simulink model "modelo_completo"  (R2020a)
settings: Solver=FixedStepAuto  StartTime=0.0  StopTime=1000.0  FixedStep=sampleTime  RelTol=1e-3
values from neighbouring files (symbols this model uses):
  FIR = [0 ... (first row only)    [Lab_3.m]
  G = 0    [Lab_3.m]
  mu = 0.03    [Lab_3.m]
  sampleTime = 0.03    [Lab_3.m]
undefined symbols (not defined in the file or in its folder): magnitude
settings Model: Creator=Gaming  LastModifiedBy=Duarte
settings SFSimCC: CustomCodeUndefinedFunction=UseInterfaceOnly

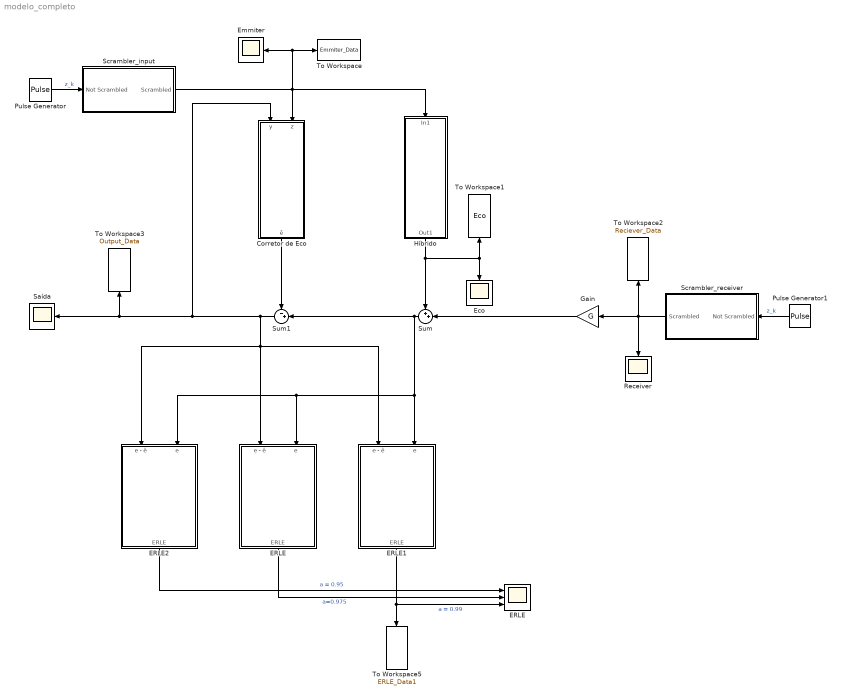
== system modelo_completo ==
  Corretor de Eco : Subsystem
  ERLE : Subsystem
  "ERLE " : Scope  NumInputPorts=3
  ERLE1 : Subsystem
  ERLE2 : Subsystem
  Eco : Scope
  Emmiter : Scope
  Gain : Gain  Gain=G
  Híbrido : Subsystem
  Pulse Generator : DiscretePulseGenerator  SampleTime=sampleTime
  Pulse Generator1 : DiscretePulseGenerator  SampleTime=sampleTime
  Receiver : Scope
  Saída : Scope
  Scrambler_input : Subsystem
  Scrambler_receiver : Subsystem
  Sum : Sum  Inputs=++|
  Sum1 : Sum  Inputs=-+|
  To Workspace : ToWorkspace  VariableName=Emmiter_Data  SaveFormat=Structure With Time  SampleTime=-1
  To Workspace1 : ToWorkspace  VariableName=Eco  SaveFormat=Structure With Time  SampleTime=-1
  To Workspace2 : ToWorkspace  VariableName=Reciever_Data  SaveFormat=Structure With Time  SampleTime=-1
  To Workspace3 : ToWorkspace  VariableName=Output_Data  SaveFormat=Structure With Time  SampleTime=-1
  To Workspace5 : ToWorkspace  VariableName=ERLE_Data1  SaveFormat=Structure With Time  SampleTime=-1
  wires:
  Pulse Generator1/1 -> Scrambler_receiver/1(Not Scrambled)  "z_k"
  Scrambler_receiver/1(Scrambled) -> Receiver/1, To Workspace2/1, Gain/1
  Gain/1 -> Sum/2
  Pulse Generator/1 -> Scrambler_input/1(Not Scrambled)  "z_k"
  Scrambler_input/1(Scrambled) -> To Workspace/1, Emmiter/1, Híbrido/1(In1), Corretor de Eco/2(z)
  Corretor de Eco/1(ê) -> Sum1/1
  Sum1/1 -> Saída/1, To Workspace3/1, Corretor de Eco/1(y), ERLE2/1(e - ê), ERLE/1(e - ê), ERLE1/1(e - ê)
  ERLE/1(ERLE) -> "ERLE "/2  "a=0.975"
  Híbrido/1(Out1) -> To Workspace1/1, Eco/1, Sum/1
  ERLE1/1(ERLE) -> "ERLE "/3, To Workspace5/1  "a = 0.99"
  ERLE2/1(ERLE) -> "ERLE "/1  "a = 0.95"
  Sum/1 -> Sum1/2, ERLE2/2(e), ERLE/2(e), ERLE1/2(e)

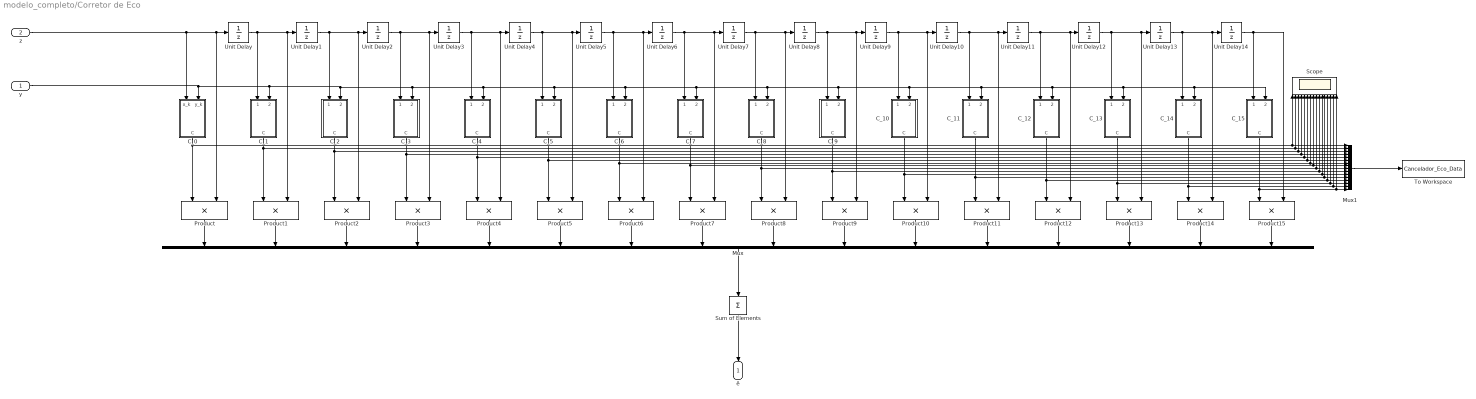
== system modelo_completo/Corretor de Eco ==
  y : Inport
  z : Inport  Port=2
  C_0 : Subsystem
  C_1 : Subsystem
  C_10 : Subsystem
  C_11 : Subsystem
  C_12 : Subsystem
  C_13 : Subsystem
  C_14 : Subsystem
  C_15 : Subsystem
  C_2 : Subsystem
  C_3 : Subsystem
  C_4 : Subsystem
  C_5 : Subsystem
  C_6 : Subsystem
  C_7 : Subsystem
  C_8 : Subsystem
  C_9 : Subsystem
  Mux : Mux  Inputs=16
  Mux1 : Mux  Inputs=16
  Product{,1..15} (16 alike) : Product
  Scope : Scope  NumInputPorts=16
  Sum of Elements : Sum  Inputs=+
  To Workspace : ToWorkspace  VariableName=Cancelador_Eco_Data  SaveFormat=Structure With Time  SampleTime=-1
  Unit Delay{,1..14} (15 alike) : UnitDelay  SampleTime=-1  HasFrameUpgradeWarning=on
  ê : Outport  VectorParamsAs1DForOutWhenUnconnected=off
  wires:
  Unit Delay9/1 -> C_10/1(x_k+1), Unit Delay10/1, Product10/2
  Unit Delay6/1 -> C_7/1(x_k+1), Unit Delay7/1, Product7/2
  C_14/1(C) -> Mux1/15, Scope/15, Product14/1
  Unit Delay8/1 -> C_9/1(x_k+1), Unit Delay9/1, Product9/2
  Product1/1 -> Mux/2
  C_13/1(C) -> Mux1/14, Scope/14, Product13/1
  Unit Delay3/1 -> C_4/1(x_k+1), Unit Delay4/1, Product4/2
  Unit Delay/1 -> Unit Delay1/1, Product1/2, C_1/1(x_k+1)
  Product13/1 -> Mux/14
  C_10/1(C) -> Mux1/11, Scope/11, Product10/1
  Unit Delay1/1 -> C_2/1(x_k+1), Unit Delay2/1, Product2/2
  Unit Delay7/1 -> C_8/1(x_k+1), Unit Delay8/1, Product8/2
  Unit Delay4/1 -> C_5/1(x_k+1), Unit Delay5/1, Product5/2
  C_9/1(C) -> Mux1/10, Scope/10, Product9/1
  Unit Delay13/1 -> C_14/1(x_k+1), Unit Delay14/1, Product14/2
  Unit Delay12/1 -> C_13/1(x_k+1), Unit Delay13/1, Product13/2
  C_11/1(C) -> Mux1/12, Scope/12, Product11/1
  Product6/1 -> Mux/7
  Unit Delay10/1 -> C_11/1(x_k+1), Unit Delay11/1, Product11/2
  C_0/1(C) -> Product/1, Mux1/1, Scope/1
  z/1 -> Unit Delay/1, Product/2, C_0/1(x_k)
  C_6/1(C) -> Mux1/7, Scope/7, Product6/1
  Unit Delay11/1 -> C_12/1(x_k+1), Unit Delay12/1, Product12/2
  C_3/1(C) -> Product3/1, Mux1/4, Scope/4
  Product15/1 -> Mux/16
  C_2/1(C) -> Product2/1, Mux1/3, Scope/3
  C_4/1(C) -> Mux1/5, Scope/5, Product4/1
  Unit Delay2/1 -> C_3/1(x_k+1), Unit Delay3/1, Product3/2
  Product4/1 -> Mux/5
  Mux/1 -> Sum of Elements/1
  Product3/1 -> Mux/4
  C_7/1(C) -> Product7/1, Mux1/8, Scope/8
  Product14/1 -> Mux/15
  Product5/1 -> Mux/6
  Product9/1 -> Mux/10
  C_1/1(C) -> Mux1/2, Scope/2, Product1/1
  Unit Delay5/1 -> C_6/1(x_k+1), Unit Delay6/1, Product6/2
  Product7/1 -> Mux/8
  Product12/1 -> Mux/13
  Product8/1 -> Mux/9
  C_8/1(C) -> Mux1/9, Scope/9, Product8/1
  Product11/1 -> Mux/12
  Product10/1 -> Mux/11
  C_15/1(C) -> Mux1/16, Scope/16, Product15/1
  Unit Delay14/1 -> C_15/1(x_k+1), Product15/2
  C_12/1(C) -> Product12/1, Mux1/13, Scope/13
  Sum of Elements/1 -> ê/1
  Product/1 -> Mux/1
  Product2/1 -> Mux/3
  Mux1/1 -> To Workspace/1
  y/1 -> C_0/2(y_k), C_7/2(y_k+1), C_11/2(y_k+1), C_14/2(y_k+1), C_15/2(y_k+1), C_13/2(y_k+1), C_12/2(y_k+1), C_10/2(y_k+1), C_9/2(y_k+1), C_8/2(y_k+1), C_6/2(y_k+1), C_5/2(y_k+1), C_4/2(y_k+1), C_3/2(y_k+1), C_2/2(y_k+1), C_1/2(y_k+1)
  C_5/1(C) -> Product5/1, Mux1/6, Scope/6

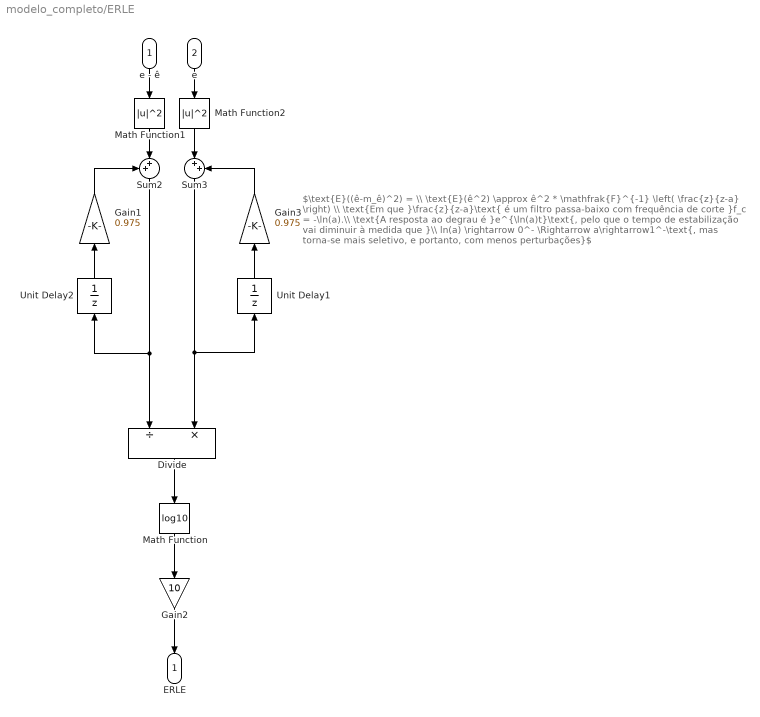
== system modelo_completo/ERLE ==
  note: $\text{E}((ê-m_ê)^2) = \\ \text{E}(ê^2) \approx ê^2 * \mathfrak{F}^{-1} \left( \frac{z}{z-a} \right) \\ \text{Em que }\frac{z}{z-a}\text{ é um filtro passa-baixo com frequência de corte }f_c = -\ln(a).\\ \text{A resposta ao degrau é }e^{\ln(a)t}\text{, pelo que o tempo de estabilização vai diminuir à medida que }\\ ln(a) \rightarrow 0^- \Rightarrow a\rightarrow1^-\text{, mas torna-se mais seletivo, e portanto, com menos perturbações}$
  e - ê : Inport
  e : Inport  Port=2
  Divide : Product  Inputs=/*
  Gain1 : Gain  Gain=0.975
  Gain2 : Gain  Gain=10
  Gain3 : Gain  Gain=0.975
  Math Function : Math  Operator=log10  SignedPower=on  SaturateOnIntegerOverflow=on
  Math Function1 : Math  Operator=magnitude^2  SignedPower=on  SaturateOnIntegerOverflow=on
  Math Function2 : Math  Operator=magnitude^2  SignedPower=on  SaturateOnIntegerOverflow=on
  Sum2 : Sum  Inputs=++|
  Sum3 : Sum  Inputs=|++
  Unit Delay1 : UnitDelay  SampleTime=-1  HasFrameUpgradeWarning=on
  Unit Delay2 : UnitDelay  SampleTime=-1  HasFrameUpgradeWarning=on
  ERLE : Outport  VectorParamsAs1DForOutWhenUnconnected=off
  wires:
  Math Function2/1 -> Sum3/1
  Math Function/1 -> Gain2/1
  Divide/1 -> Math Function/1
  Unit Delay2/1 -> Gain1/1
  Unit Delay1/1 -> Gain3/1
  e - ê/1 -> Math Function1/1
  Sum3/1 -> Divide/2, Unit Delay1/1
  Gain3/1 -> Sum3/2
  Math Function1/1 -> Sum2/2
  Sum2/1 -> Unit Delay2/1, Divide/1
  Gain1/1 -> Sum2/1
  e/1 -> Math Function2/1
  Gain2/1 -> ERLE/1

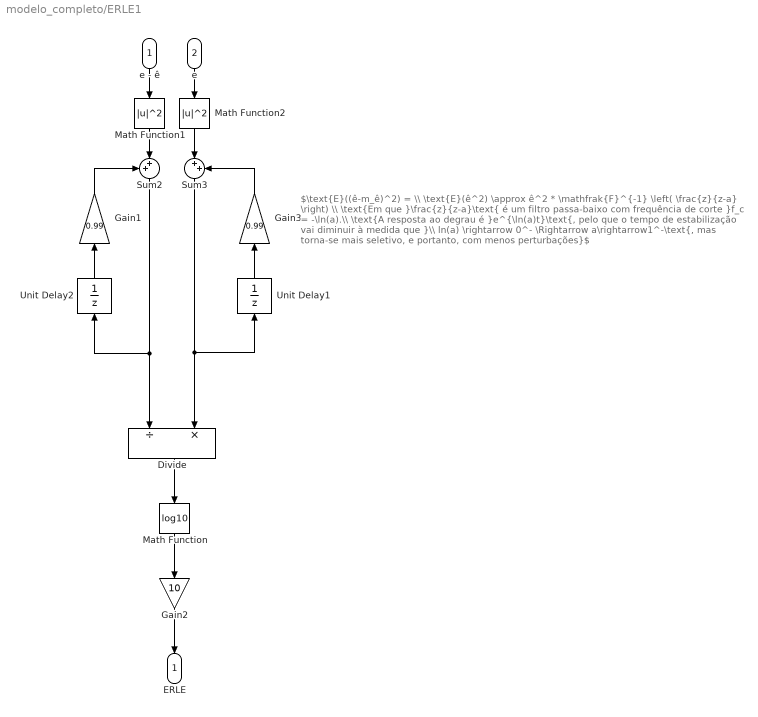
== system modelo_completo/ERLE1 ==
  note: $\text{E}((ê-m_ê)^2) = \\ \text{E}(ê^2) \approx ê^2 * \mathfrak{F}^{-1} \left( \frac{z}{z-a} \right) \\ \text{Em que }\frac{z}{z-a}\text{ é um filtro passa-baixo com frequência de corte }f_c = -\ln(a).\\ \text{A resposta ao degrau é }e^{\ln(a)t}\text{, pelo que o tempo de estabilização vai diminuir à medida que }\\ ln(a) \rightarrow 0^- \Rightarrow a\rightarrow1^-\text{, mas torna-se mais seletivo, e portanto, com menos perturbações}$
  e - ê : Inport
  e : Inport  Port=2
  Divide : Product  Inputs=/*
  Gain1 : Gain  Gain=0.99
  Gain2 : Gain  Gain=10
  Gain3 : Gain  Gain=0.99
  Math Function : Math  Operator=log10  SignedPower=on  SaturateOnIntegerOverflow=on
  Math Function1 : Math  Operator=magnitude^2  SignedPower=on  SaturateOnIntegerOverflow=on
  Math Function2 : Math  Operator=magnitude^2  SignedPower=on  SaturateOnIntegerOverflow=on
  Sum2 : Sum  Inputs=++|
  Sum3 : Sum  Inputs=|++
  Unit Delay1 : UnitDelay  SampleTime=-1  HasFrameUpgradeWarning=on
  Unit Delay2 : UnitDelay  SampleTime=-1  HasFrameUpgradeWarning=on
  ERLE : Outport  VectorParamsAs1DForOutWhenUnconnected=off
  wires:
  Math Function2/1 -> Sum3/1
  Math Function/1 -> Gain2/1
  Divide/1 -> Math Function/1
  Unit Delay2/1 -> Gain1/1
  Unit Delay1/1 -> Gain3/1
  e - ê/1 -> Math Function1/1
  Sum3/1 -> Divide/2, Unit Delay1/1
  Gain3/1 -> Sum3/2
  Math Function1/1 -> Sum2/2
  Sum2/1 -> Unit Delay2/1, Divide/1
  Gain1/1 -> Sum2/1
  e/1 -> Math Function2/1
  Gain2/1 -> ERLE/1

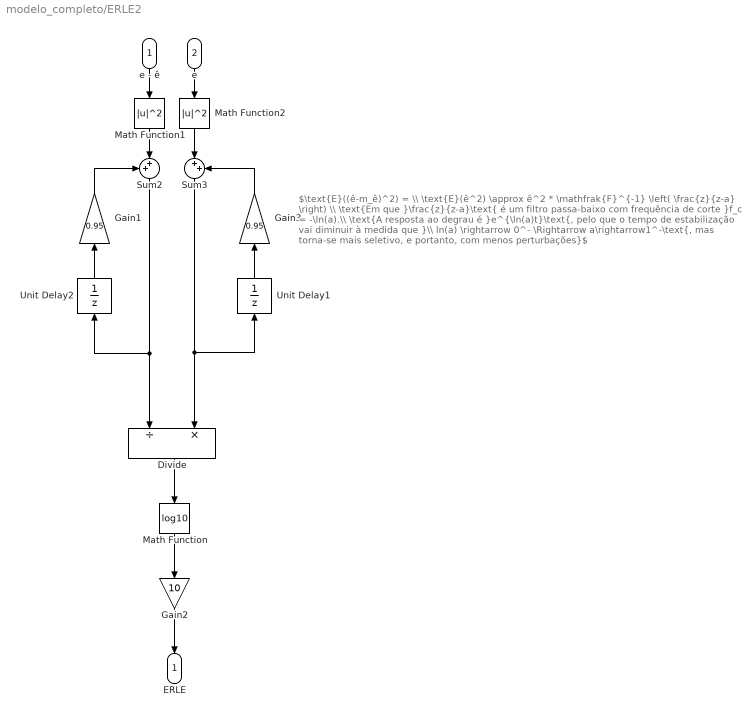
== system modelo_completo/ERLE2 ==
  note: $\text{E}((ê-m_ê)^2) = \\ \text{E}(ê^2) \approx ê^2 * \mathfrak{F}^{-1} \left( \frac{z}{z-a} \right) \\ \text{Em que }\frac{z}{z-a}\text{ é um filtro passa-baixo com frequência de corte }f_c = -\ln(a).\\ \text{A resposta ao degrau é }e^{\ln(a)t}\text{, pelo que o tempo de estabilização vai diminuir à medida que }\\ ln(a) \rightarrow 0^- \Rightarrow a\rightarrow1^-\text{, mas torna-se mais seletivo, e portanto, com menos perturbações}$
  e - ê : Inport
  e : Inport  Port=2
  Divide : Product  Inputs=/*
  Gain1 : Gain  Gain=0.95
  Gain2 : Gain  Gain=10
  Gain3 : Gain  Gain=0.95
  Math Function : Math  Operator=log10  SignedPower=on  SaturateOnIntegerOverflow=on
  Math Function1 : Math  Operator=magnitude^2  SignedPower=on  SaturateOnIntegerOverflow=on
  Math Function2 : Math  Operator=magnitude^2  SignedPower=on  SaturateOnIntegerOverflow=on
  Sum2 : Sum  Inputs=++|
  Sum3 : Sum  Inputs=|++
  Unit Delay1 : UnitDelay  SampleTime=-1  HasFrameUpgradeWarning=on
  Unit Delay2 : UnitDelay  SampleTime=-1  HasFrameUpgradeWarning=on
  ERLE : Outport  VectorParamsAs1DForOutWhenUnconnected=off
  wires:
  Math Function2/1 -> Sum3/1
  Math Function/1 -> Gain2/1
  Divide/1 -> Math Function/1
  Unit Delay2/1 -> Gain1/1
  Unit Delay1/1 -> Gain3/1
  e - ê/1 -> Math Function1/1
  Sum3/1 -> Divide/2, Unit Delay1/1
  Gain3/1 -> Sum3/2
  Math Function1/1 -> Sum2/2
  Sum2/1 -> Unit Delay2/1, Divide/1
  Gain1/1 -> Sum2/1
  e/1 -> Math Function2/1
  Gain2/1 -> ERLE/1

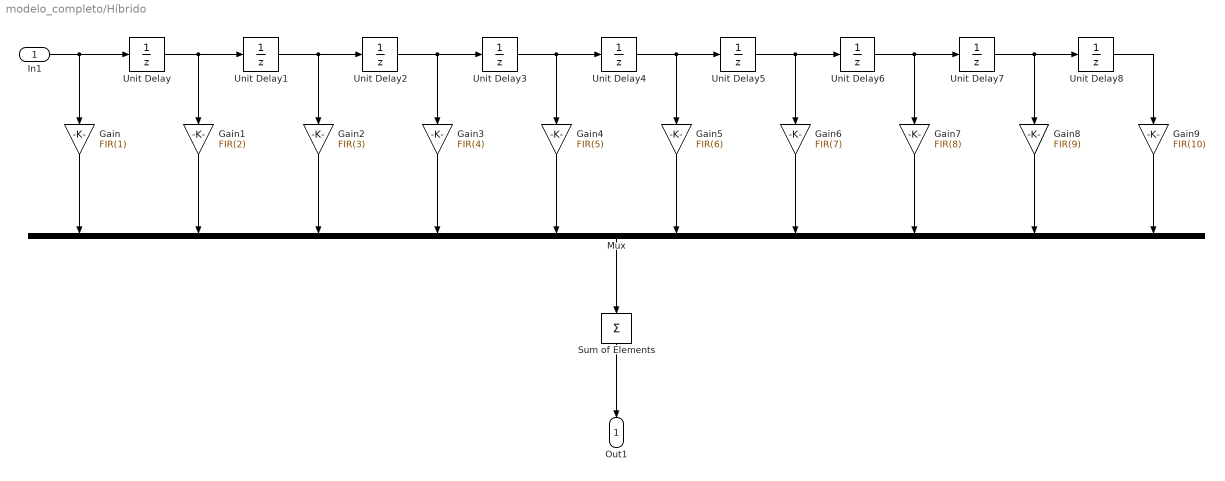
== system modelo_completo/Híbrido ==
  In1 : Inport
  Gain : Gain  Gain=FIR(1)
  Gain1 : Gain  Gain=FIR(2)
  Gain2 : Gain  Gain=FIR(3)
  Gain3 : Gain  Gain=FIR(4)
  Gain4 : Gain  Gain=FIR(5)
  Gain5 : Gain  Gain=FIR(6)
  Gain6 : Gain  Gain=FIR(7)
  Gain7 : Gain  Gain=FIR(8)
  Gain8 : Gain  Gain=FIR(9)
  Gain9 : Gain  Gain=FIR(10)
  Mux : Mux  Inputs=10
  Sum of Elements : Sum  Inputs=+
  Unit Delay{,1..8} (9 alike) : UnitDelay  SampleTime=-1  HasFrameUpgradeWarning=on
  Out1 : Outport  VectorParamsAs1DForOutWhenUnconnected=off
  wires:
  Unit Delay1/1 -> Gain2/1, Unit Delay2/1
  In1/1 -> Unit Delay/1, Gain/1
  Unit Delay/1 -> Unit Delay1/1, Gain1/1
  Unit Delay2/1 -> Gain3/1, Unit Delay3/1
  Unit Delay7/1 -> Gain8/1, Unit Delay8/1
  Unit Delay8/1 -> Gain9/1
  Unit Delay5/1 -> Unit Delay6/1, Gain6/1
  Unit Delay6/1 -> Gain7/1, Unit Delay7/1
  Unit Delay4/1 -> Unit Delay5/1, Gain5/1
  Unit Delay3/1 -> Unit Delay4/1, Gain4/1
  Mux/1 -> Sum of Elements/1
  Sum of Elements/1 -> Out1/1
  Gain/1 -> Mux/1
  Gain1/1 -> Mux/2
  Gain9/1 -> Mux/10
  Gain8/1 -> Mux/9
  Gain7/1 -> Mux/8
  Gain6/1 -> Mux/7
  Gain5/1 -> Mux/6
  Gain4/1 -> Mux/5
  Gain3/1 -> Mux/4
  Gain2/1 -> Mux/3

== system modelo_completo/Scrambler_input ==
  Not Scrambled : Inport
  Bias : Bias  Bias=-1
  Delay : Delay  DelayLength=3
  Delay1 : Delay
  Gain : Gain  Gain=2  OutDataTypeStr=double
  XOR : Logic  Operator=XOR  Inputs=3  AllPortsSameDT=off  OutDataTypeStr=boolean
  Scrambled : Outport  VectorParamsAs1DForOutWhenUnconnected=off
  wires:
  Bias/1 -> Scrambled/1
  Gain/1 -> Bias/1
  Not Scrambled/1 -> XOR/1
  Delay/1 -> Delay1/1, XOR/3
  Delay1/1 -> XOR/2
  XOR/1 -> Delay/1, Gain/1

== system modelo_completo/Scrambler_receiver ==
  Not Scrambled : Inport
  Bias : Bias  Bias=-1
  Delay : Delay  DelayLength=5
  Delay1 : Delay
  Gain : Gain  Gain=2  OutDataTypeStr=double
  XOR : Logic  Operator=XOR  Inputs=3  AllPortsSameDT=off  OutDataTypeStr=boolean
  Scrambled : Outport  VectorParamsAs1DForOutWhenUnconnected=off
  wires:
  Gain/1 -> Bias/1
  XOR/1 -> Delay/1, Gain/1
  Delay/1 -> XOR/3, Delay1/1
  Not Scrambled/1 -> XOR/1
  Delay1/1 -> XOR/2
  Bias/1 -> Scrambled/1

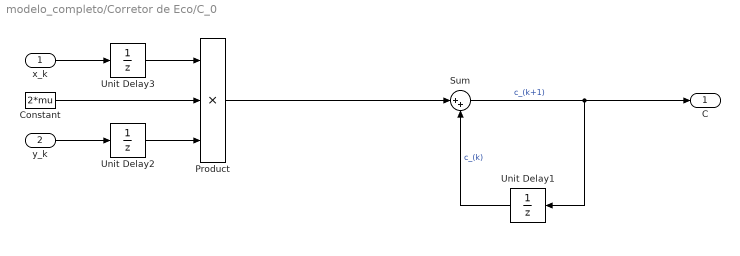
== system modelo_completo/Corretor de Eco/C_0 ==
  x_k : Inport
  y_k : Inport  Port=2
  Constant : Constant  Value=2*mu
  Product : Product  Inputs=3
  Sum : Sum  Inputs=|++
  Unit Delay1 : UnitDelay  SampleTime=-1  HasFrameUpgradeWarning=on
  Unit Delay2 : UnitDelay  SampleTime=-1  HasFrameUpgradeWarning=on
  Unit Delay3 : UnitDelay  SampleTime=-1  HasFrameUpgradeWarning=on
  C : Outport  VectorParamsAs1DForOutWhenUnconnected=off
  wires:
  x_k/1 -> Unit Delay3/1
  y_k/1 -> Unit Delay2/1
  Product/1 -> Sum/1
  Constant/1 -> Product/2
  Unit Delay1/1 -> Sum/2  "c_(k)"
  Sum/1 -> Unit Delay1/1, C/1  "c_(k+1)"
  Unit Delay2/1 -> Product/3
  Unit Delay3/1 -> Product/1

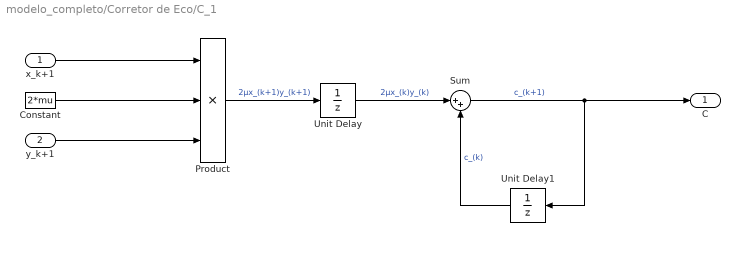
== system modelo_completo/Corretor de Eco/C_1 ==
  x_k+1 : Inport
  y_k+1 : Inport  Port=2
  Constant : Constant  Value=2*mu
  Product : Product  Inputs=3
  Sum : Sum  Inputs=|++
  Unit Delay : UnitDelay  SampleTime=-1  HasFrameUpgradeWarning=on
  Unit Delay1 : UnitDelay  SampleTime=-1  HasFrameUpgradeWarning=on
  C : Outport  VectorParamsAs1DForOutWhenUnconnected=off
  wires:
  x_k+1/1 -> Product/1
  y_k+1/1 -> Product/3
  Product/1 -> Unit Delay/1  "2μx_(k+1)y_(k+1)"
  Constant/1 -> Product/2
  Unit Delay/1 -> Sum/1  "2μx_(k)y_(k)"
  Unit Delay1/1 -> Sum/2  "c_(k)"
  Sum/1 -> Unit Delay1/1, C/1  "c_(k+1)"

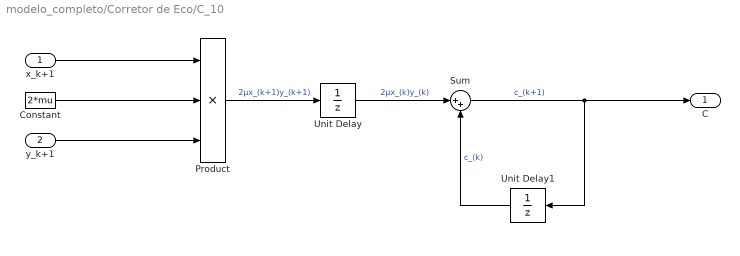
== system modelo_completo/Corretor de Eco/C_10 ==
  x_k+1 : Inport
  y_k+1 : Inport  Port=2
  Constant : Constant  Value=2*mu
  Product : Product  Inputs=3
  Sum : Sum  Inputs=|++
  Unit Delay : UnitDelay  SampleTime=-1  HasFrameUpgradeWarning=on
  Unit Delay1 : UnitDelay  SampleTime=-1  HasFrameUpgradeWarning=on
  C : Outport  VectorParamsAs1DForOutWhenUnconnected=off
  wires:
  x_k+1/1 -> Product/1
  y_k+1/1 -> Product/3
  Product/1 -> Unit Delay/1  "2μx_(k+1)y_(k+1)"
  Constant/1 -> Product/2
  Unit Delay/1 -> Sum/1  "2μx_(k)y_(k)"
  Unit Delay1/1 -> Sum/2  "c_(k)"
  Sum/1 -> Unit Delay1/1, C/1  "c_(k+1)"

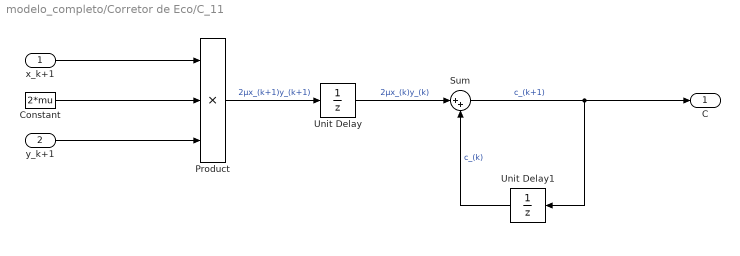
== system modelo_completo/Corretor de Eco/C_11 ==
  x_k+1 : Inport
  y_k+1 : Inport  Port=2
  Constant : Constant  Value=2*mu
  Product : Product  Inputs=3
  Sum : Sum  Inputs=|++
  Unit Delay : UnitDelay  SampleTime=-1  HasFrameUpgradeWarning=on
  Unit Delay1 : UnitDelay  SampleTime=-1  HasFrameUpgradeWarning=on
  C : Outport  VectorParamsAs1DForOutWhenUnconnected=off
  wires:
  x_k+1/1 -> Product/1
  y_k+1/1 -> Product/3
  Product/1 -> Unit Delay/1  "2μx_(k+1)y_(k+1)"
  Constant/1 -> Product/2
  Unit Delay/1 -> Sum/1  "2μx_(k)y_(k)"
  Unit Delay1/1 -> Sum/2  "c_(k)"
  Sum/1 -> Unit Delay1/1, C/1  "c_(k+1)"

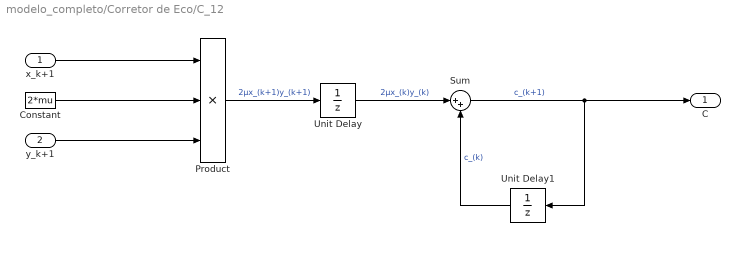
== system modelo_completo/Corretor de Eco/C_12 ==
  x_k+1 : Inport
  y_k+1 : Inport  Port=2
  Constant : Constant  Value=2*mu
  Product : Product  Inputs=3
  Sum : Sum  Inputs=|++
  Unit Delay : UnitDelay  SampleTime=-1  HasFrameUpgradeWarning=on
  Unit Delay1 : UnitDelay  SampleTime=-1  HasFrameUpgradeWarning=on
  C : Outport  VectorParamsAs1DForOutWhenUnconnected=off
  wires:
  x_k+1/1 -> Product/1
  y_k+1/1 -> Product/3
  Product/1 -> Unit Delay/1  "2μx_(k+1)y_(k+1)"
  Constant/1 -> Product/2
  Unit Delay/1 -> Sum/1  "2μx_(k)y_(k)"
  Unit Delay1/1 -> Sum/2  "c_(k)"
  Sum/1 -> Unit Delay1/1, C/1  "c_(k+1)"

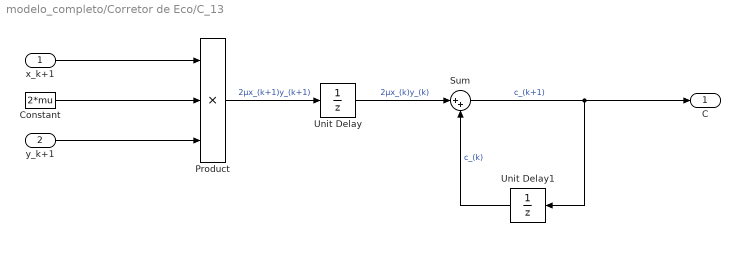
== system modelo_completo/Corretor de Eco/C_13 ==
  x_k+1 : Inport
  y_k+1 : Inport  Port=2
  Constant : Constant  Value=2*mu
  Product : Product  Inputs=3
  Sum : Sum  Inputs=|++
  Unit Delay : UnitDelay  SampleTime=-1  HasFrameUpgradeWarning=on
  Unit Delay1 : UnitDelay  SampleTime=-1  HasFrameUpgradeWarning=on
  C : Outport  VectorParamsAs1DForOutWhenUnconnected=off
  wires:
  x_k+1/1 -> Product/1
  y_k+1/1 -> Product/3
  Product/1 -> Unit Delay/1  "2μx_(k+1)y_(k+1)"
  Constant/1 -> Product/2
  Unit Delay/1 -> Sum/1  "2μx_(k)y_(k)"
  Unit Delay1/1 -> Sum/2  "c_(k)"
  Sum/1 -> Unit Delay1/1, C/1  "c_(k+1)"

== system modelo_completo/Corretor de Eco/C_14 ==
  x_k+1 : Inport
  y_k+1 : Inport  Port=2
  Constant : Constant  Value=2*mu
  Product : Product  Inputs=3
  Sum : Sum  Inputs=|++
  Unit Delay : UnitDelay  SampleTime=-1  HasFrameUpgradeWarning=on
  Unit Delay1 : UnitDelay  SampleTime=-1  HasFrameUpgradeWarning=on
  C : Outport  VectorParamsAs1DForOutWhenUnconnected=off
  wires:
  x_k+1/1 -> Product/1
  y_k+1/1 -> Product/3
  Product/1 -> Unit Delay/1  "2μx_(k+1)y_(k+1)"
  Constant/1 -> Product/2
  Unit Delay/1 -> Sum/1  "2μx_(k)y_(k)"
  Unit Delay1/1 -> Sum/2  "c_(k)"
  Sum/1 -> Unit Delay1/1, C/1  "c_(k+1)"

== system modelo_completo/Corretor de Eco/C_15 ==
  x_k+1 : Inport
  y_k+1 : Inport  Port=2
  Constant : Constant  Value=2*mu
  Product : Product  Inputs=3
  Sum : Sum  Inputs=|++
  Unit Delay : UnitDelay  SampleTime=-1  HasFrameUpgradeWarning=on
  Unit Delay1 : UnitDelay  SampleTime=-1  HasFrameUpgradeWarning=on
  C : Outport  VectorParamsAs1DForOutWhenUnconnected=off
  wires:
  x_k+1/1 -> Product/1
  y_k+1/1 -> Product/3
  Product/1 -> Unit Delay/1  "2μx_(k+1)y_(k+1)"
  Constant/1 -> Product/2
  Unit Delay/1 -> Sum/1  "2μx_(k)y_(k)"
  Unit Delay1/1 -> Sum/2  "c_(k)"
  Sum/1 -> Unit Delay1/1, C/1  "c_(k+1)"

== system modelo_completo/Corretor de Eco/C_2 ==
  x_k+1 : Inport
  y_k+1 : Inport  Port=2
  Constant : Constant  Value=2*mu
  Product : Product  Inputs=3
  Sum : Sum  Inputs=|++
  Unit Delay : UnitDelay  SampleTime=-1  HasFrameUpgradeWarning=on
  Unit Delay1 : UnitDelay  SampleTime=-1  HasFrameUpgradeWarning=on
  C : Outport  VectorParamsAs1DForOutWhenUnconnected=off
  wires:
  x_k+1/1 -> Product/1
  y_k+1/1 -> Product/3
  Product/1 -> Unit Delay/1  "2μx_(k+1)y_(k+1)"
  Constant/1 -> Product/2
  Unit Delay/1 -> Sum/1  "2μx_(k)y_(k)"
  Unit Delay1/1 -> Sum/2  "c_(k)"
  Sum/1 -> Unit Delay1/1, C/1  "c_(k+1)"

== system modelo_completo/Corretor de Eco/C_3 ==
  x_k+1 : Inport
  y_k+1 : Inport  Port=2
  Constant : Constant  Value=2*mu
  Product : Product  Inputs=3
  Sum : Sum  Inputs=|++
  Unit Delay : UnitDelay  SampleTime=-1  HasFrameUpgradeWarning=on
  Unit Delay1 : UnitDelay  SampleTime=-1  HasFrameUpgradeWarning=on
  C : Outport  VectorParamsAs1DForOutWhenUnconnected=off
  wires:
  x_k+1/1 -> Product/1
  y_k+1/1 -> Product/3
  Product/1 -> Unit Delay/1  "2μx_(k+1)y_(k+1)"
  Constant/1 -> Product/2
  Unit Delay/1 -> Sum/1  "2μx_(k)y_(k)"
  Unit Delay1/1 -> Sum/2  "c_(k)"
  Sum/1 -> Unit Delay1/1, C/1  "c_(k+1)"

== system modelo_completo/Corretor de Eco/C_4 ==
  x_k+1 : Inport
  y_k+1 : Inport  Port=2
  Constant : Constant  Value=2*mu
  Product : Product  Inputs=3
  Sum : Sum  Inputs=|++
  Unit Delay : UnitDelay  SampleTime=-1  HasFrameUpgradeWarning=on
  Unit Delay1 : UnitDelay  SampleTime=-1  HasFrameUpgradeWarning=on
  C : Outport  VectorParamsAs1DForOutWhenUnconnected=off
  wires:
  x_k+1/1 -> Product/1
  y_k+1/1 -> Product/3
  Product/1 -> Unit Delay/1  "2μx_(k+1)y_(k+1)"
  Constant/1 -> Product/2
  Unit Delay/1 -> Sum/1  "2μx_(k)y_(k)"
  Unit Delay1/1 -> Sum/2  "c_(k)"
  Sum/1 -> Unit Delay1/1, C/1  "c_(k+1)"

== system modelo_completo/Corretor de Eco/C_5 ==
  x_k+1 : Inport
  y_k+1 : Inport  Port=2
  Constant : Constant  Value=2*mu
  Product : Product  Inputs=3
  Sum : Sum  Inputs=|++
  Unit Delay : UnitDelay  SampleTime=-1  HasFrameUpgradeWarning=on
  Unit Delay1 : UnitDelay  SampleTime=-1  HasFrameUpgradeWarning=on
  C : Outport  VectorParamsAs1DForOutWhenUnconnected=off
  wires:
  x_k+1/1 -> Product/1
  y_k+1/1 -> Product/3
  Product/1 -> Unit Delay/1  "2μx_(k+1)y_(k+1)"
  Constant/1 -> Product/2
  Unit Delay/1 -> Sum/1  "2μx_(k)y_(k)"
  Unit Delay1/1 -> Sum/2  "c_(k)"
  Sum/1 -> Unit Delay1/1, C/1  "c_(k+1)"

== system modelo_completo/Corretor de Eco/C_6 ==
  x_k+1 : Inport
  y_k+1 : Inport  Port=2
  Constant : Constant  Value=2*mu
  Product : Product  Inputs=3
  Sum : Sum  Inputs=|++
  Unit Delay : UnitDelay  SampleTime=-1  HasFrameUpgradeWarning=on
  Unit Delay1 : UnitDelay  SampleTime=-1  HasFrameUpgradeWarning=on
  C : Outport  VectorParamsAs1DForOutWhenUnconnected=off
  wires:
  x_k+1/1 -> Product/1
  y_k+1/1 -> Product/3
  Product/1 -> Unit Delay/1  "2μx_(k+1)y_(k+1)"
  Constant/1 -> Product/2
  Unit Delay/1 -> Sum/1  "2μx_(k)y_(k)"
  Unit Delay1/1 -> Sum/2  "c_(k)"
  Sum/1 -> Unit Delay1/1, C/1  "c_(k+1)"

== system modelo_completo/Corretor de Eco/C_7 ==
  x_k+1 : Inport
  y_k+1 : Inport  Port=2
  Constant : Constant  Value=2*mu
  Product : Product  Inputs=3
  Sum : Sum  Inputs=|++
  Unit Delay : UnitDelay  SampleTime=-1  HasFrameUpgradeWarning=on
  Unit Delay1 : UnitDelay  SampleTime=-1  HasFrameUpgradeWarning=on
  C : Outport  VectorParamsAs1DForOutWhenUnconnected=off
  wires:
  x_k+1/1 -> Product/1
  y_k+1/1 -> Product/3
  Product/1 -> Unit Delay/1  "2μx_(k+1)y_(k+1)"
  Constant/1 -> Product/2
  Unit Delay/1 -> Sum/1  "2μx_(k)y_(k)"
  Unit Delay1/1 -> Sum/2  "c_(k)"
  Sum/1 -> Unit Delay1/1, C/1  "c_(k+1)"

== system modelo_completo/Corretor de Eco/C_8 ==
  x_k+1 : Inport
  y_k+1 : Inport  Port=2
  Constant : Constant  Value=2*mu
  Product : Product  Inputs=3
  Sum : Sum  Inputs=|++
  Unit Delay : UnitDelay  SampleTime=-1  HasFrameUpgradeWarning=on
  Unit Delay1 : UnitDelay  SampleTime=-1  HasFrameUpgradeWarning=on
  C : Outport  VectorParamsAs1DForOutWhenUnconnected=off
  wires:
  x_k+1/1 -> Product/1
  y_k+1/1 -> Product/3
  Product/1 -> Unit Delay/1  "2μx_(k+1)y_(k+1)"
  Constant/1 -> Product/2
  Unit Delay/1 -> Sum/1  "2μx_(k)y_(k)"
  Unit Delay1/1 -> Sum/2  "c_(k)"
  Sum/1 -> Unit Delay1/1, C/1  "c_(k+1)"

== system modelo_completo/Corretor de Eco/C_9 ==
  x_k+1 : Inport
  y_k+1 : Inport  Port=2
  Constant : Constant  Value=2*mu
  Product : Product  Inputs=3
  Sum : Sum  Inputs=|++
  Unit Delay : UnitDelay  SampleTime=-1  HasFrameUpgradeWarning=on
  Unit Delay1 : UnitDelay  SampleTime=-1  HasFrameUpgradeWarning=on
  C : Outport  VectorParamsAs1DForOutWhenUnconnected=off
  wires:
  x_k+1/1 -> Product/1
  y_k+1/1 -> Product/3
  Product/1 -> Unit Delay/1  "2μx_(k+1)y_(k+1)"
  Constant/1 -> Product/2
  Unit Delay/1 -> Sum/1  "2μx_(k)y_(k)"
  Unit Delay1/1 -> Sum/2  "c_(k)"
  Sum/1 -> Unit Delay1/1, C/1  "c_(k+1)"
